simulink model "speed_esc_closed_loop"  (R2022b)
settings: Solver=FixedStepDiscrete  StartTime=0.0  StopTime=119.90000000000001  FixedStep=0.10000000000000001  RelTol=1e-3
InitFcn:
  | addpath(fileparts(fileparts(get_param(bdroot,'FileName'))));
model workspace (MAT data in the model file):
  noise_input = [0 0.1 0.2 0.3 0.4 0.5 0.6 0.7 0.8 0.9 1 1.1 ... (2400 elements, 1200x2)]
  private_optimum_input = [0 0.1 0.2 0.3 0.4 0.5 0.6 0.7 0.8 0.9 1 1.1 ... (2400 elements, 1200x2)]
  speed_configuration.version = 3
  speed_configuration.curve = 'cubic'
  speed_configuration.method = 'regression'
  speed_configuration.mode = 'esc'
  speed_configuration.Ts = 0.1
  speed_configuration.duration = 120
  speed_configuration.initialSpeed = 10
  speed_configuration.lower = 0
  speed_configuration.upper = 20
  speed_configuration.tau = 2
  speed_configuration.noiseSigma = 0.02
  speed_configuration.delay = 0.5
  speed_configuration.seed = 1
  speed_configuration.shift = 1
  speed_configuration.shiftTime = 60
  speed_configuration.optimum = 6.3
  speed_configuration.shiftedOptimum = 9
  speed_configuration.minimumRatio = 0.913
  speed_configuration.amplitude = 0.5
  speed_configuration.omega = 0.5
  speed_configuration.gain = 8
  speed_configuration.hpOmega = 0.1
  speed_configuration.lpOmega = 2
  speed_configuration.window = 126
  speed_configuration.minimumSpeedStd = 0.025
  speed_configuration.gradientLimit = 1
  speed_configuration.centerRate = 0.8
  speed_configuration.referenceRate = 1
  speed_configuration.maxAge = 2
  speed_configuration.fixedReference = 10
  speed_configuration.tailSeconds = 20
  speed_configuration.settlingWindow = 12.6
  speed_configuration.settlingHold = 5
  speed_configuration.rlPeriod = 1
  valid_input = [0 0.1 0.2 0.3 0.4 0.5 0.6 0.7 0.8 0.9 1 1.1 ... (2400 elements, 1200x2)]
(part 1 of 2)
settings Model: Creator=偷走月亮的猫  LastModifiedBy=偷走月亮的猫

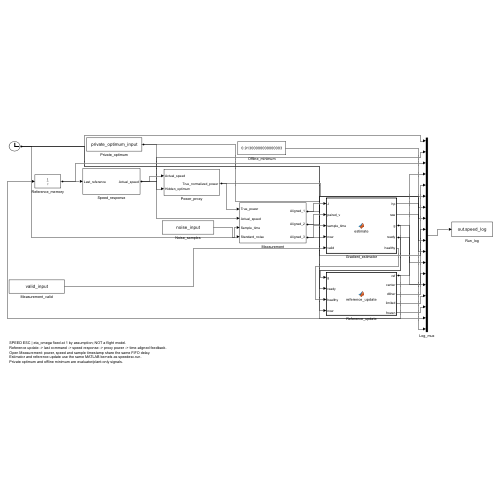
[thumbnail: Simulink's stored preview of the top-level diagram]
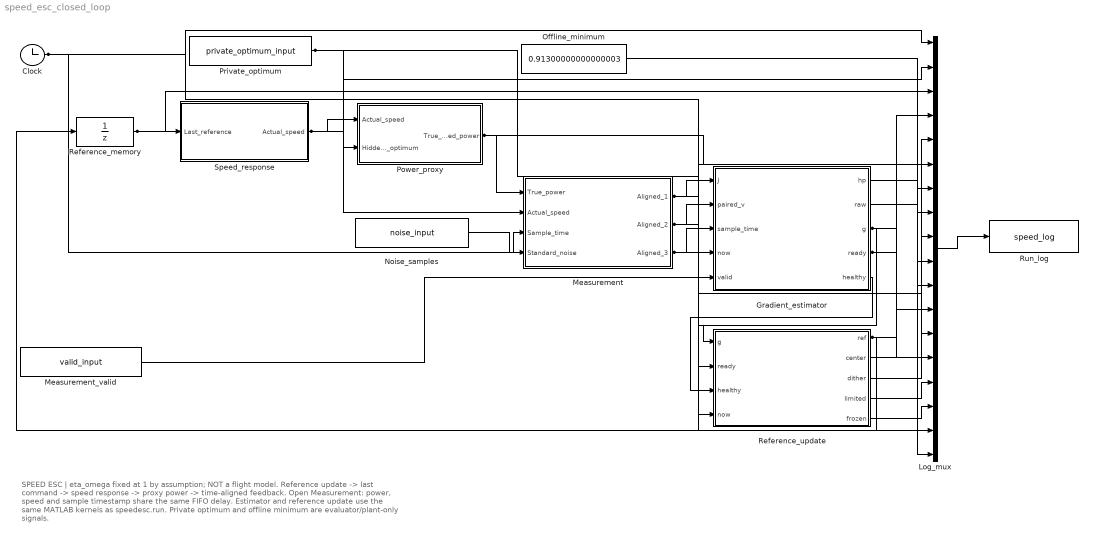
== system speed_esc_closed_loop ==
  note: SPEED ESC | eta_omega fixed at 1 by assumption; NOT a flight model.
      | Reference update -> last command -> speed response -> proxy power -> time-aligned feedback.
      | Open Measurement: power, speed and sample timestamp share the same FIFO delay.
      | Estimator and reference update use the same MATLAB kernels as speedesc.run.
      | Private optimum and offline minimum are evaluator/plant-only signals.
  Clock : Clock
  Gradient_estimator : MATLAB Function  TreatAsAtomicUnit=on
  Log_mux : Mux  Inputs=18
  Measurement : Subsystem
  Measurement_valid : FromWorkspace  VariableName=valid_input  Interpolate=off  OutputAfterFinalValue=Holding final value
  Noise_samples : FromWorkspace  VariableName=noise_input  Interpolate=off  OutputAfterFinalValue=Holding final value
  Offline_minimum : Constant  Value=0.91300000000000003
  Power_proxy : Subsystem
  Private_optimum : FromWorkspace  VariableName=private_optimum_input  Interpolate=off  OutputAfterFinalValue=Holding final value
  Reference_memory : UnitDelay  InitialCondition=10  SampleTime=0.10000000000000001  HasFrameUpgradeWarning=on
  Reference_update : MATLAB Function  TreatAsAtomicUnit=on
  Run_log : ToWorkspace  VariableName=speed_log  SampleTime=-1
  Speed_response : Subsystem
  wires:
  Reference_memory/1 -> Speed_response/1(Last_reference), Log_mux/3
  Speed_response/1(Actual_speed) -> Power_proxy/1(Actual_speed), Measurement/2(Actual_speed), Log_mux/2
  Private_optimum/1 -> Power_proxy/2(Hidden_optimum), Log_mux/17
  Power_proxy/1(True_normalized_power) -> Measurement/1(True_power), Log_mux/6
  Clock/1 -> Measurement/3(Sample_time), Gradient_estimator/4(now), Reference_update/4(now), Log_mux/1
  Noise_samples/1 -> Measurement/4(Standard_noise)
  Measurement/1(Aligned_1) -> Gradient_estimator/1(J), Log_mux/7
  Measurement/2(Aligned_2) -> Gradient_estimator/2(paired_v), Log_mux/8
  Measurement/3(Aligned_3) -> Gradient_estimator/3(sample_time), Log_mux/9
  Measurement_valid/1 -> Gradient_estimator/5(valid)
  Gradient_estimator/3(g) -> Reference_update/1(g), Log_mux/12
  Gradient_estimator/4(ready) -> Reference_update/2(ready), Log_mux/14
  Gradient_estimator/5(healthy) -> Reference_update/3(healthy)
  Reference_update/1(ref) -> Reference_memory/1, Log_mux/4
  Reference_update/2(center) -> Log_mux/5
  Gradient_estimator/1(hp) -> Log_mux/10
  Gradient_estimator/2(raw) -> Log_mux/11
  Reference_update/3(dither) -> Log_mux/13
  Reference_update/4(limited) -> Log_mux/15
  Reference_update/5(frozen) -> Log_mux/16
  Offline_minimum/1 -> Log_mux/18
  Log_mux/1 -> Run_log/1
